simulink model "q_3d_crane"  (Simulink 6.6)
settings: Solver=FixedStepDiscrete  StartTime=0.0  StopTime=inf  FixedStep=0.001  RelTol=1e-3
StopFcn:
  | callback_clear_setpoints
values from neighbouring files (symbols this model uses):
  ALPHA_LIM_ENABLE = 1    [setup_3d_crane.m]
  ALPHA_MAX = 25    [setup_3d_crane.m]
  ALPHA_MIN = - ALPHA_MAX    (= -25)    [setup_3d_crane.m]
  GAMMA_LIM_ENABLE = 1    [setup_3d_crane.m]
  GAMMA_MAX = 25    [setup_3d_crane.m]
  GAMMA_MIN = - GAMMA_MAX    (= -25)    [setup_3d_crane.m]
  IMAX_AMP = 7    [setup_3d_crane.m]
  K_CURR = -2.0    (= -2)    [config_3d_crane.m]
  K_ENC_ALPHA = 2 * pi / (4 * 1024 )    (= 0.00153398078789)    [config_3d_crane.m]
  K_ENC_GAMMA = 2 * pi / (4 * 1024 )    (= 0.00153398078789)    [config_3d_crane.m]
  K_ENC_THETA = 2 * pi / (4 * 1024 ) / Kg_t    (= 1.53398078789e-05)    [config_3d_crane.m]
  K_ENC_X = - Pt / (4 * 1024 ) / Kg_j    [config_3d_crane.m]
  K_ENC_Z = - 2 * pi * r_y_reel / (4 * 1024 ) / Kg_y    [config_3d_crane.m]
  K_J = lqr(A_J,B_J,Q_J,R_J)    [setup_3d_crane.m]
  K_T = lqr(A_T,B_T,Q_T,R_T)    [setup_3d_crane.m]
  Ka = 0.5    [config_3d_crane.m]
  ki = w0^2*p0*(mp*r_y_reel^2+J_phi)/eff_g_y/Kg_y/eff_m_y/Kt_y/r_y_reel    [d_payload_piv_controller.m]
  kp = w0*(2*zeta*p0*J_phi+w0*mp*r_y_reel^2+w0*J_phi+2*zeta*p0*mp*r_y_reel^2)/eff_g_y/Kg_y/eff_m_y/Kt_y/r_y_reel    [d_payload_piv_controller.m]
  kv = (p0*J_phi+2*zeta*w0*mp*r_y_reel^2+2*zeta*w0*J_phi+p0*mp*r_y_reel^2)/eff_g_y/Kg_y/eff_m_y/Kt_y/r_y_reel    [d_payload_piv_controller.m]
  LS_LIM_ENABLE = 1    [setup_3d_crane.m]
  VMAX_DAC = 10    [setup_3d_crane.m]
  wf_gamma = 2 * pi * 2.0    (= 12.5663706144)    [setup_3d_crane.m]
  wf_theta = 2 * pi * 50    (= 314.159265359)    [setup_3d_crane.m]
  wf_x = 2 * pi * 50    (= 314.159265359)    [setup_3d_crane.m]
  wf_z = 2 * pi * 50    (= 314.159265359)    [setup_3d_crane.m]
  X_LIM_ENABLE = 1    [setup_3d_crane.m]
  X_MAX = 0.4    [setup_3d_crane.m]
  X_MIN = - X_MAX    (= -0.4)    [setup_3d_crane.m]
  Z_LIM_ENABLE = 1    [setup_3d_crane.m]
  Z_MAX = 0.7    [setup_3d_crane.m]
  Z_MIN = -0.05    [setup_3d_crane.m]
undefined symbols (not defined in the file or in its folder): DiscIntNeverNeededParam, HIL, qc_get_step_size
libraries: quarc_library x28, simulink x13, simulink_extras x6
settings Model: Creator=MLevis  LastModifiedBy=MLevis  SimulationMode=external  ExtModeTrigDuration=25000
settings SolverCC: PositivePriorityOrder=on
settings RTWCC: SystemTargetFile=quarc_windows.tlc  TemplateMakefile=quarc_default_tmf  Description=QuaRC Win32 Target  ProcessScript=quarc_windows_make_rtw_hook
settings STFCustomTargetCC: TargetFcnLib=ansi_tfl_tmw.mat  TargetPreCompLibLocation=C:\DOCUME~1\ALLUSE~1\APPLIC~1\QUARC\lib\2007a\windows\release  GenFloatMathFcnCalls=ANSI_C  SystemTargetFile=quarc_windows.tlc
settings GRTTargetCC: TargetPreCompLibLocation=C:\DOCUME~1\ALLUSE~1\APPLIC~1\QUARC\lib\2007a\windows\release  MatFileLogging=off  ExtMode=on  ExtModeMexFile=quarc_comm

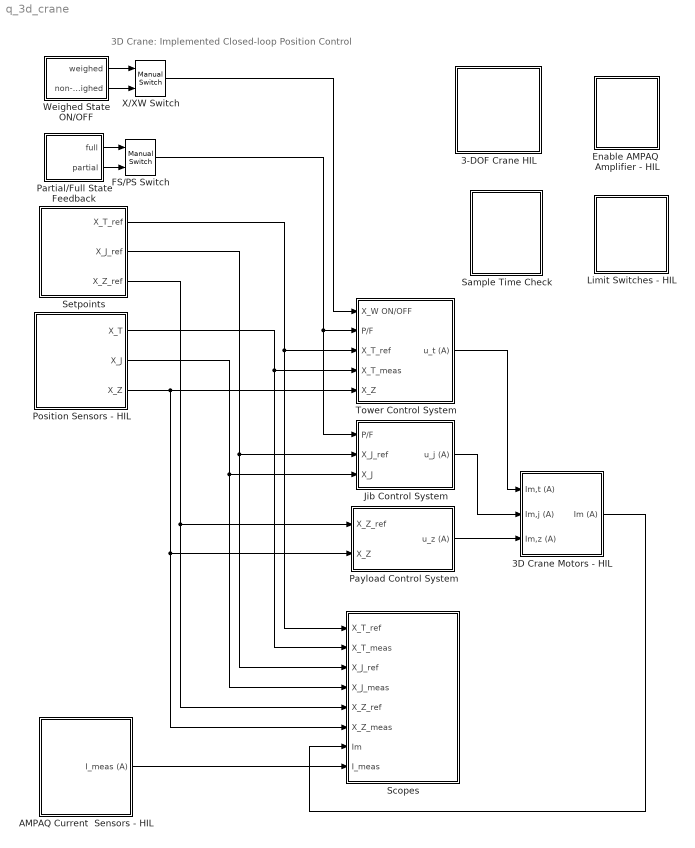
== system q_3d_crane ==
  note: 3D Crane: Implemented Closed-loop Position Control
  3-DOF Crane HIL : Subsystem
  3D Crane Motors - HIL : Subsystem
  AMPAQ Current  Sensors - HIL : Subsystem
  Enable AMPAQ  Amplifier - HIL : Subsystem
  FS/PS Switch : simulink/Signal Routing/Manual Switch  SystemSampleTime=-1  sw=1  action=0  varsize=off
  Jib Control System : Subsystem
  Limit Switches - HIL : Subsystem
  Partial/Full State Feedback : Subsystem
  Payload Control System : Subsystem
  Position Sensors - HIL : Subsystem
  Sample Time Check : Subsystem
  Scopes : Subsystem
  Setpoints : Subsystem
  Tower Control System : Subsystem
  Weighed State ON/OFF : Subsystem
  X/XW Switch : simulink/Signal Routing/Manual Switch  SystemSampleTime=-1  sw=1  action=0  varsize=off
  wires:
  Payload Control System/1(u_z (A)) -> 3D Crane Motors - HIL/3(Im,z (A))
  Tower Control System/1(u_t (A)) -> 3D Crane Motors - HIL/1(Im,t (A))
  Position Sensors - HIL/1(X_T) -> Scopes/2(X_T_meas), Tower Control System/4(X_T_meas)
  Position Sensors - HIL/3(X_Z) -> Scopes/6(X_Z_meas), Payload Control System/2(X_Z), Tower Control System/5(X_Z)
  Position Sensors - HIL/2(X_J) -> Scopes/4(X_J_meas), Jib Control System/3(X_J)
  Setpoints/2(X_J_ref) -> Scopes/3(X_J_ref), Jib Control System/2(X_J_ref)
  Setpoints/1(X_T_ref) -> Scopes/1(X_T_ref), Tower Control System/3(X_T_ref)
  Setpoints/3(X_Z_ref) -> Scopes/5(X_Z_ref), Payload Control System/1(X_Z_ref)
  Jib Control System/1(u_j (A)) -> 3D Crane Motors - HIL/2(Im,j (A))
  Partial/Full State Feedback/1(full) -> FS/PS Switch/1
  Partial/Full State Feedback/2(partial) -> FS/PS Switch/2
  Weighed State ON/OFF/1(weighed) -> X/XW Switch/1
  Weighed State ON/OFF/2(non-weighed) -> X/XW Switch/2
  X/XW Switch/1 -> Tower Control System/1(X_W ON/OFF)
  FS/PS Switch/1 -> Tower Control System/2(P/F), Jib Control System/1(P/F)
  3D Crane Motors - HIL/1(Im (A)) -> Scopes/7(Im)
  AMPAQ Current  Sensors - HIL/1(I_meas (A)) -> Scopes/8(I_meas)

== system q_3d_crane/3-DOF Crane HIL ==
  HIL Initialize : quarc_library/Data Acquisition/Generic/Configuration/HIL Initialize  object_name=HIL-1  board_type=q8  board_number=0  exclusive=off  active=on  hardware_clocks=[0:1]  clock_modes=[0 0]  initial_clock_frequencies=[]  set_clock_params_at_start=on  set_clock_params_at_switch_in=off  set_clock_frequencies_at_start=off  set_clock_frequencies_at_switch_in=off  analog_input_channels=[0:7]  analog_input_maximums=10  analog_input_minimums=-10  set_analog_input_params_at_start=off  set_analog_input_params_at_switch_in=off  analog_output_channels=[0:7]  analog_output_maximums=[10]  analog_output_minimums=[-10]  initial_analog_outputs=[0]  final_analog_outputs=[0]  watchdog_analog_outputs=0  set_analog_output_params_at_start=on  set_analog_output_params_at_switch_in=off  set_analog_outputs_at_start=on  set_analog_outputs_at_switch_in=off  set_analog_outputs_at_terminate=on  set_analog_outputs_at_switch_out=off  set_analog_outputs_on_watchdog=off  digital_input_channels=[]  digital_output_channels=[0:2,4]  digital_output_configuration=[]  initial_digital_outputs=[1]  final_digital_outputs=[1]  watchdog_digital_outputs=[2]  set_digital_output_params_at_start=off  set_digital_output_params_at_switch_in=off  set_digital_outputs_at_start=on  set_digital_outputs_at_switch_in=off  set_digital_outputs_at_terminate=on  set_digital_outputs_at_switch_out=off  set_digital_outputs_on_watchdog=off  encoder_channels=[0:7]  quadrature=[4]  encoder_filter_frequency=(1/120e-9)/1  initial_encoder_counts=[0]  set_encoder_params_at_start=on  set_encoder_params_at_switch_in=off  set_encoder_counts_at_start=on  set_encoder_counts_at_switch_in=off  pwm_channels=[]  pwm_modes=[0]  pwm_frequency=(1/60e-9)/1024  pwm_configuration=[]  pwm_alignment=[]  pwm_polarity=[]  pwm_leading_deadband=[]  pwm_trailing_deadband=[]  initial_pwm_outputs=[0]  final_pwm_outputs=[0]  watchdog_pwm_outputs=[]  set_pwm_params_at_start=on  set_pwm_params_at_switch_in=off  set_pwm_outputs_at_start=on  set_pwm_outputs_at_switch_in=off  set_pwm_outputs_at_terminate=on  set_pwm_outputs_at_switch_out=off  set_pwm_outputs_on_watchdog=off  other_output_channels=[]  initial_other_outputs=[]  final_other_outputs=[]  watchdog_other_outputs=[]  set_other_outputs_at_start=off  set_other_outputs_at_switch_in=off  set_other_outputs_at_terminate=off  set_other_outputs_at_switch_out=off  set_other_outputs_on_watchdog=off
      settings: AttributesFormatString=%<object_name>
  HIL Read Timebase : quarc_library/Data Acquisition/Generic/Timebases/HIL Read Timebase  Tag=unassigned  object_name=HIL-1  clock=0  analog_channels=[0:2]  encoder_channels=[0:4]  digital_channels=[8:12]  other_channels=[]  samples_in_buffer=max(ceil(1/qc_get_step_size), 1)  active=on  vector_output=on  data_type_mode=Inherit via back propagation  encoder_data_type=double  digital_data_type=boolean
  HIL Write : quarc_library/Data Acquisition/Generic/Immediate I//O/HIL Write  Tag=unassigned  object_name=HIL-1  analog_channels=[0:2]  pwm_channels=[]  digital_channels=[0:2,4]  other_channels=[]  sample_time=-1  active=off  vector_input=on
  tag scope: AI=global, DI=global, ENC_CNT=global
  wires:
  HIL Read Timebase/3 -> [DI]
  HIL Read Timebase/1 -> [AI]
  HIL Read Timebase/2 -> [ENC_CNT]
  [DO] -> HIL Write/2
  [AO] -> HIL Write/1

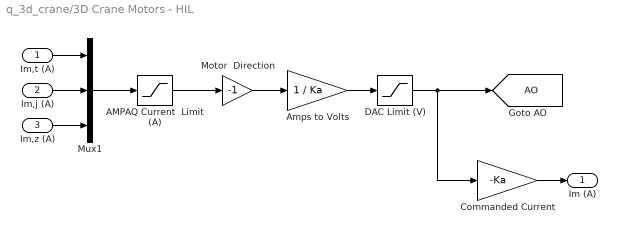
== system q_3d_crane/3D Crane Motors - HIL ==
  Im,t (A) : Inport
  Im,j (A) : Inport  Port=2
  Im,z (A) : Inport  Port=3
  AMPAQ Current  Limit (A) : Saturate  UpperLimit=IMAX_AMP  LowerLimit=-IMAX_AMP
  Amps to Volts : Gain  Gain=1 / Ka  SaturateOnIntegerOverflow=on
  "Commanded Current " : Gain  Gain=-Ka  SaturateOnIntegerOverflow=on
  DAC Limit (V) : Saturate  UpperLimit=VMAX_DAC  LowerLimit=-VMAX_DAC
  Motor  Direction : Gain  Gain=-1
  Mux1 : Mux  Inputs=3
  Im (A) : Outport
  tag scope: AO=global
  wires:
  Amps to Volts/1 -> DAC Limit (V)/1
  DAC Limit (V)/1 -> [AO], "Commanded Current "/1
  AMPAQ Current  Limit (A)/1 -> Motor  Direction/1
  Im,t (A)/1 -> Mux1/1
  Im,j (A)/1 -> Mux1/2
  Im,z (A)/1 -> Mux1/3
  Mux1/1 -> AMPAQ Current  Limit (A)/1
  "Commanded Current "/1 -> Im (A)/1
  Motor  Direction/1 -> Amps to Volts/1

== system q_3d_crane/AMPAQ Current  Sensors - HIL ==
  note: AMPAQ Current Sensors
  Current Sensitivity (A/V) : Gain  Gain=K_CURR
  I_meas (A) : Outport
  wires:
  Current Sensitivity (A/V)/1 -> I_meas (A)/1
  [AI] -> Current Sensitivity (A/V)/1

== system q_3d_crane/Enable AMPAQ  Amplifier - HIL ==
  Enable Amp : Constant  Value=[0 0 0 1]
  tag scope: DO=global
  wires:
  Enable Amp/1 -> [DO]

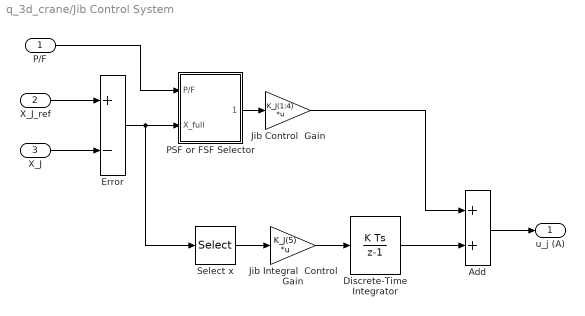
== system q_3d_crane/Jib Control System ==
  P/F : Inport
  X_J_ref : Inport  Port=2
  X_J : Inport  Port=3
  Add : Sum  OutScaling=2^-10
  Discrete-Time Integrator : DiscreteIntegrator  SampleTime=qc_get_step_size  LimitOutput=on  UpperSaturationLimit=2  LowerSaturationLimit=-2  ICPrevOutput=DiscIntNeverNeededParam  ICPrevScaledInput=DiscIntNeverNeededParam
  Error : Sum  Inputs=+-  OutScaling=2^-10
  Jib Control  Gain : Gain  Gain=K_J(1:4)  Multiplication=Matrix(K*u)
  Jib Integral  Control Gain : Gain  Gain=K_J(5)  Multiplication=Matrix(K*u)
  PSF or FSF Selector : Subsystem
  Select x : Selector  IndexOptions=Index vector (dialog)  Indices=1  OutputSizes=1  InputPortWidth=4
  u_j (A) : Outport
  wires:
  PSF or FSF Selector/1(X_out) -> Jib Control  Gain/1
  P/F/1 -> PSF or FSF Selector/1(P/F)
  Add/1 -> u_j (A)/1
  Discrete-Time Integrator/1 -> Add/2
  Jib Control  Gain/1 -> Add/1
  Jib Integral  Control Gain/1 -> Discrete-Time Integrator/1
  Select x/1 -> Jib Integral  Control Gain/1
  X_J/1 -> Error/2
  X_J_ref/1 -> Error/1
  Error/1 -> Select x/1, PSF or FSF Selector/2(X_full)

== system q_3d_crane/Limit Switches - HIL ==
  Constant3 : Constant  Orientation=down  Value=LS_LIM_ENABLE
  Read Limit Switches : Subsystem
  Stop with Limit Switches : Subsystem  TreatAsAtomicUnit=on
  wires:
  Constant3/1 -> Stop with Limit Switches/Enable
  Read Limit Switches/1(tower cw) -> Stop with Limit Switches/1(tower cw)
  Read Limit Switches/2(tower ccw) -> Stop with Limit Switches/2(tower ccw)
  Read Limit Switches/3(jib ret) -> Stop with Limit Switches/3(jib ret)
  Read Limit Switches/4(jib ext) -> Stop with Limit Switches/4(jib ext)
  Read Limit Switches/5(payload max) -> Stop with Limit Switches/5(payload max)

== system q_3d_crane/Partial/Full State Feedback ==
  Full-State : Constant
  Partial-State : Constant  Value=0
  full : Outport
  partial : Outport  Port=2
  wires:
  Full-State/1 -> full/1
  Partial-State/1 -> partial/1

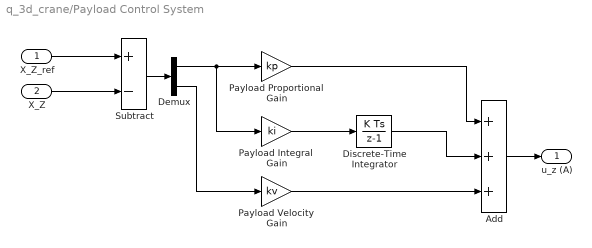
== system q_3d_crane/Payload Control System ==
  X_Z_ref : Inport
  X_Z : Inport  Port=2
  Add : Sum  Inputs=+++  OutScaling=2^-10
  Demux : Demux  Outputs=2
  Discrete-Time Integrator : DiscreteIntegrator  SampleTime=qc_get_step_size  ICPrevOutput=DiscIntNeverNeededParam  ICPrevScaledInput=DiscIntNeverNeededParam
  Payload Integral  Gain : Gain  Gain=ki
  Payload Proportional  Gain : Gain  Gain=kp
  Payload Velocity  Gain : Gain  Gain=kv
  Subtract : Sum  Inputs=+-  OutScaling=2^-10
  u_z (A) : Outport
  wires:
  X_Z/1 -> Subtract/2
  X_Z_ref/1 -> Subtract/1
  Payload Integral  Gain/1 -> Discrete-Time Integrator/1
  Add/1 -> u_z (A)/1
  Payload Proportional  Gain/1 -> Add/1
  Discrete-Time Integrator/1 -> Add/2
  Subtract/1 -> Demux/1
  Demux/1 -> Payload Proportional  Gain/1, Payload Integral  Gain/1
  Demux/2 -> Payload Velocity  Gain/1
  Payload Velocity  Gain/1 -> Add/3

== system q_3d_crane/Position Sensors - HIL ==
  note: 3D Crane Encoders
  Construct Jib State : Subsystem
  Construct Payload State : Subsystem
  Construct Tower State : Subsystem
  Encoder Calibration : Gain  Gain=[K_ENC_THETA, K_ENC_X, K_ENC_Z, K_ENC_ALPHA, K_ENC_GAMMA]
  X_T : Outport
  X_J : Outport  Port=2
  X_Z : Outport  Port=3
  wires:
  [ENC_CNT] -> Encoder Calibration/1
  Encoder Calibration/1 -> Construct Tower State/1(X_read), Construct Jib State/1(X_read), Construct Payload State/1(X_read)
  Construct Tower State/1(X_T) -> X_T/1
  Construct Jib State/1(X_J) -> X_J/1
  Construct Payload State/1(X_Z) -> X_Z/1

== system q_3d_crane/Sample Time Check ==
  Larger than  2x sample time? : simulink/Logic and Bit Operations/Compare To Constant  SystemSampleTime=-1  relop=>  const=2*qc_get_step_size  LogicOutDataTypeMode=uint8  ZeroCross=off
  Max Missed Samples : simulink/Logic and Bit Operations/Compare To Constant  SystemSampleTime=-1  relop=>  const=5  LogicOutDataTypeMode=uint8  ZeroCross=off
  Memory : Memory  Orientation=left
  Sample Time : quarc_library/Sources/Time/Sample Time  Priority=-99  sample_time=qc_get_step_size
  Samples Missed : Display
  Stop with Message : quarc_library/Sinks/Error Handling/Stop with Message  SystemSampleTime=-1  message_type=Fixed error message  message_icon=Error  message=Maximum number of missed samples reached. Please reduce your CPU load.
  Sum : Sum  Inputs=|++
  wires:
  Max Missed Samples/1 -> Stop with Message/1
  Memory/1 -> Sum/2
  Sum/1 -> Memory/1, Max Missed Samples/1, Samples Missed/1
  Larger than  2x sample time?/1 -> Sum/1
  Sample Time/1 -> Larger than  2x sample time?/1

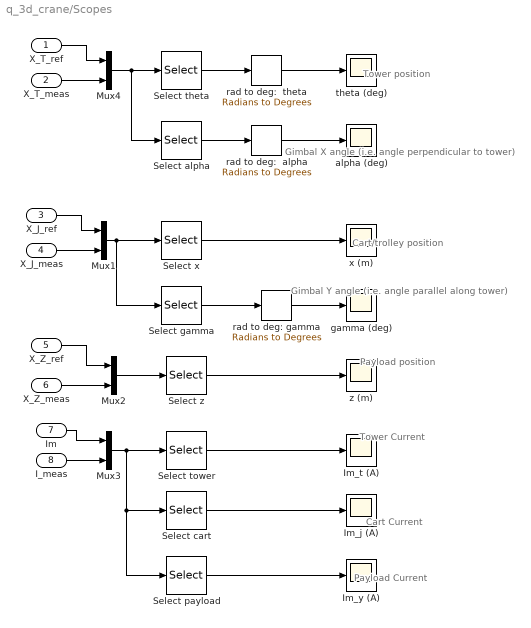
== system q_3d_crane/Scopes ==
  note: Tower Current
  note: Cart Current
  note: Payload Current
  note: Payload position
  note: Cart/trolley position
  note: Tower position
  note: Gimbal X angle
      | (i.e. angle perpendicular to tower)
  note: Gimbal Y angle
      | (i.e. angle parallel along tower)
  X_T_ref : Inport
  X_T_meas : Inport  Port=2
  X_J_ref : Inport  Port=3
  X_J_meas : Inport  Port=4
  X_Z_ref : Inport  Port=5
  X_Z_meas : Inport  Port=6
  Im : Inport  Port=7
  I_meas : Inport  Port=8
  Im_j (A) : Scope
      settings: TimeRange=25  SaveName=ScopeData4
  Im_t (A) : Scope
      settings: TimeRange=25  SaveName=ScopeData3
  Im_y (A) : Scope
      settings: TimeRange=25  SaveName=ScopeData5
  Mux{1..4} (4 alike) : Mux  Inputs=2
  Select alpha : Selector  IndexOptions=Index vector (dialog)  Indices=[2 6]  OutputSizes=1  InputPortWidth=8
  Select cart : Selector  IndexOptions=Index vector (dialog)  Indices=[2 5]  OutputSizes=1  InputPortWidth=6
  Select gamma : Selector  IndexOptions=Index vector (dialog)  Indices=[2 6]  OutputSizes=1  InputPortWidth=8
  Select payload : Selector  IndexOptions=Index vector (dialog)  Indices=[3 6]  OutputSizes=1  InputPortWidth=6
  Select theta : Selector  IndexOptions=Index vector (dialog)  Indices=[1 5]  OutputSizes=1  InputPortWidth=8
  Select tower : Selector  IndexOptions=Index vector (dialog)  Indices=[1 4]  OutputSizes=1  InputPortWidth=6
  Select x : Selector  IndexOptions=Index vector (dialog)  Indices=[1 5]  OutputSizes=1  InputPortWidth=8
  Select z : Selector  IndexOptions=Index vector (dialog)  Indices=[1 3]  OutputSizes=1  InputPortWidth=4
  alpha (deg) : Scope
      settings: TimeRange=25  YMin=-15  YMax=15
  gamma (deg) : Scope
      settings: TimeRange=25  SaveName=ScopeData9
  rad to deg:  theta : simulink_extras/Transformations/Radians to Degrees  SystemSampleTime=-1
  rad to deg: gamma : simulink_extras/Transformations/Radians to Degrees  SystemSampleTime=-1
  rad to deg:  alpha : simulink_extras/Transformations/Radians to Degrees  SystemSampleTime=-1
  theta (deg) : Scope
      settings: TimeRange=25  YMin=-150  YMax=150  SaveName=ScopeData8
  x (m) : Scope
      settings: TimeRange=25  YMin=-1  YMax=1
  z (m) : Scope
      settings: TimeRange=25  YMin=0  YMax=0.65  SaveName=ScopeData2
  wires:
  I_meas/1 -> Mux3/2
  Mux3/1 -> Select tower/1, Select payload/1, Select cart/1
  Im/1 -> Mux3/1
  rad to deg:  theta/1 -> theta (deg)/1
  rad to deg: gamma/1 -> gamma (deg)/1
  rad to deg:  alpha/1 -> alpha (deg)/1
  Select theta/1 -> rad to deg:  theta/1
  X_T_ref/1 -> Mux4/1
  Mux4/1 -> Select theta/1, Select alpha/1
  Select x/1 -> x (m)/1
  Mux2/1 -> Select z/1
  Select alpha/1 -> rad to deg:  alpha/1
  Select gamma/1 -> rad to deg: gamma/1
  X_J_ref/1 -> Mux1/1
  X_J_meas/1 -> Mux1/2
  Mux1/1 -> Select x/1, Select gamma/1
  X_Z_ref/1 -> Mux2/1
  X_Z_meas/1 -> Mux2/2
  Select z/1 -> z (m)/1
  X_T_meas/1 -> Mux4/2
  Select tower/1 -> Im_t (A)/1
  Select cart/1 -> Im_j (A)/1
  Select payload/1 -> Im_y (A)/1

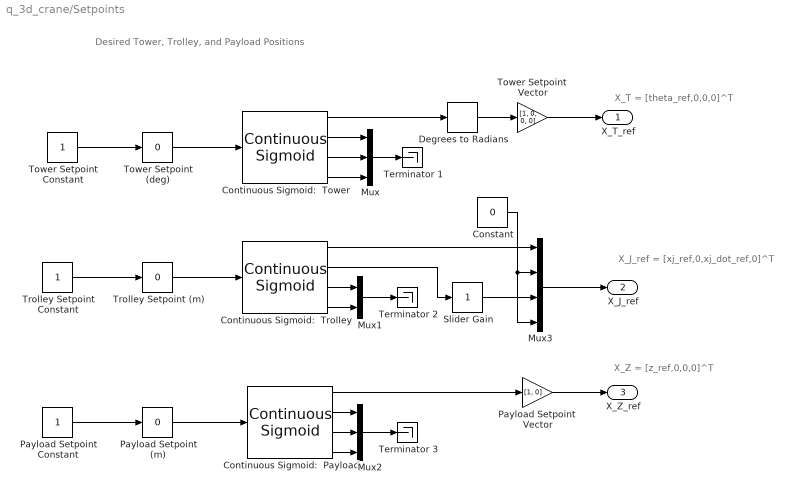
== system q_3d_crane/Setpoints ==
  note: X_J_ref = [xj_ref,0,xj_dot_ref,0]^T
  note: X_T = [theta_ref,0,0,0]^T
  note: X_Z = [z_ref,0,0,0]^T
  note: Desired Tower, Trolley, and Payload Positions
  Constant : Constant  Value=0
  Continuous Sigmoid:  Payload : quarc_library/Sources/Sigmoids/Continuous Sigmoid  params_source=Internal (dialog parameters)  max_velocity=0.25  max_acceleration=0.25  initial_position=0  initial_velocity=0  hold_off=0.5  input_sample_time=-1  output_sample_time=qc_get_step_size
  Continuous Sigmoid:  Tower : quarc_library/Sources/Sigmoids/Continuous Sigmoid  params_source=Internal (dialog parameters)  max_velocity=75  max_acceleration=45  initial_position=0  initial_velocity=0  hold_off=0.5  input_sample_time=-1  output_sample_time=qc_get_step_size
  Continuous Sigmoid:  Trolley : quarc_library/Sources/Sigmoids/Continuous Sigmoid  params_source=Internal (dialog parameters)  max_velocity=0.75  max_acceleration=1.5  initial_position=0  initial_velocity=0  hold_off=0.5  input_sample_time=-1  output_sample_time=qc_get_step_size
  Degrees to Radians : simulink_extras/Transformations/Degrees to Radians  SystemSampleTime=-1
  Mux : Mux  Inputs=3
  Mux1 : Mux  Inputs=2
  Mux2 : Mux  Inputs=3
  Mux3 : Mux
  "Payload Setpoint Constant " : Constant
  Payload Setpoint  Vector : Gain  Gain=[1, 0]
  Payload Setpoint (m) : simulink/Math Operations/Slider Gain  SystemSampleTime=-1  low=0  gain=0  high=0.8
  Slider Gain : simulink/Math Operations/Slider Gain  SystemSampleTime=-1  low=0  gain=1  high=1
  Terminator 1 : Terminator
  Terminator 2 : Terminator
  Terminator 3 : Terminator
  "Tower Setpoint Constant " : Constant
  Tower Setpoint  Vector : Gain  Gain=[1, 0, 0, 0]
  Tower Setpoint (deg) : simulink/Math Operations/Slider Gain  SystemSampleTime=-1  low=-120  gain=0  high=120
  "Trolley Setpoint Constant " : Constant
  Trolley Setpoint (m) : simulink/Math Operations/Slider Gain  SystemSampleTime=-1  low=-0.2  gain=0  high=0.2
  X_T_ref : Outport
  X_J_ref : Outport  Port=2
  X_Z_ref : Outport  Port=3
  wires:
  Continuous Sigmoid:  Tower/1 -> Degrees to Radians/1
  "Tower Setpoint Constant "/1 -> Tower Setpoint (deg)/1
  Tower Setpoint (deg)/1 -> Continuous Sigmoid:  Tower/1
  "Trolley Setpoint Constant "/1 -> Trolley Setpoint (m)/1
  "Payload Setpoint Constant "/1 -> Payload Setpoint (m)/1
  Degrees to Radians/1 -> Tower Setpoint  Vector/1
  Continuous Sigmoid:  Tower/2 -> Mux/1
  Continuous Sigmoid:  Tower/3 -> Mux/2
  Continuous Sigmoid:  Tower/4 -> Mux/3
  Mux/1 -> Terminator 1/1
  Payload Setpoint (m)/1 -> Continuous Sigmoid:  Payload/1
  Tower Setpoint  Vector/1 -> X_T_ref/1
  Continuous Sigmoid:  Payload/1 -> Payload Setpoint  Vector/1
  Payload Setpoint  Vector/1 -> X_Z_ref/1
  Trolley Setpoint (m)/1 -> Continuous Sigmoid:  Trolley/1
  Mux3/1 -> X_J_ref/1
  Continuous Sigmoid:  Trolley/1 -> Mux3/1
  Constant/1 -> Mux3/2, Mux3/4
  Continuous Sigmoid:  Trolley/2 -> Slider Gain/1
  Slider Gain/1 -> Mux3/3
  Mux1/1 -> Terminator 2/1
  Mux2/1 -> Terminator 3/1
  Continuous Sigmoid:  Payload/2 -> Mux2/1
  Continuous Sigmoid:  Payload/3 -> Mux2/2
  Continuous Sigmoid:  Payload/4 -> Mux2/3
  Continuous Sigmoid:  Trolley/3 -> Mux1/1
  Continuous Sigmoid:  Trolley/4 -> Mux1/2

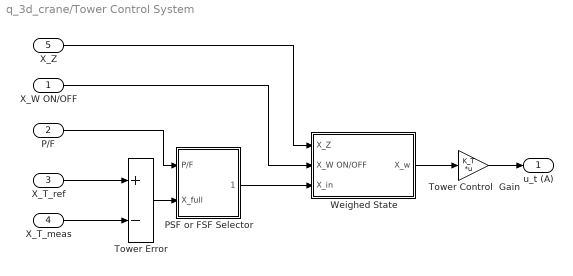
== system q_3d_crane/Tower Control System ==
  X_W ON/OFF : Inport
  P/F : Inport  Port=2
  X_T_ref : Inport  Port=3
  X_T_meas : Inport  Port=4
  X_Z : Inport  Port=5
  PSF or FSF Selector : Subsystem
  Tower Control  Gain : Gain  Gain=K_T  Multiplication=Matrix(K*u)
  Tower Error : Sum  Inputs=+-  OutScaling=2^-10
  Weighed State : Subsystem
  u_t (A) : Outport
  wires:
  Tower Control  Gain/1 -> u_t (A)/1
  X_T_ref/1 -> Tower Error/1
  X_T_meas/1 -> Tower Error/2
  P/F/1 -> PSF or FSF Selector/1(P/F)
  Tower Error/1 -> PSF or FSF Selector/2(X_full)
  X_Z/1 -> Weighed State/1(X_Z)
  X_W ON/OFF/1 -> Weighed State/2(X_W ON/OFF)
  PSF or FSF Selector/1(X_out) -> Weighed State/3(X_in)
  Weighed State/1(X_w) -> Tower Control  Gain/1

== system q_3d_crane/Weighed State ON/OFF ==
  Full State : Constant  Value=0
  Weighed State : Constant
  weighed : Outport
  non-weighed : Outport  Port=2
  wires:
  Weighed State/1 -> weighed/1
  Full State/1 -> non-weighed/1

== system q_3d_crane/Jib Control System/PSF or FSF Selector ==
  note: Partial-state or Full-state Feedback
  note: 0 = partial and 1 = full,
  note: state
  note: control input
  P/F : Inport
  X_full : Inport  Port=2
  Constant: FS : Constant  Value=[1 1 1 1]
  Constant: PS : Constant  Value=[1 0 1 0]
  Full-state : Product  RndMeth=Zero
  Multiport Switch : MultiPortSwitch  Inputs=2  zeroidx=on
  Partial-state : Product  RndMeth=Zero
  X_out : Outport
  wires:
  Constant: FS/1 -> Full-state/2
  Constant: PS/1 -> Partial-state/1
  Partial-state/1 -> Multiport Switch/2
  Full-state/1 -> Multiport Switch/3
  Multiport Switch/1 -> X_out/1
  P/F/1 -> Multiport Switch/1
  X_full/1 -> Partial-state/2, Full-state/1

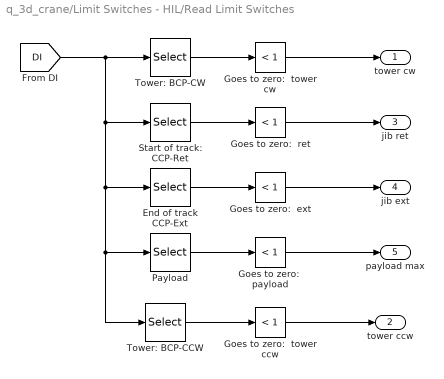
== system q_3d_crane/Limit Switches - HIL/Read Limit Switches ==
  End of track CCP-Ext : Selector  IndexOptions=Index vector (dialog)  Indices=3  OutputSizes=1  InputPortWidth=5
  Goes to zero:  ext : simulink/Logic and Bit Operations/Compare To Constant  SystemSampleTime=-1  relop=<  const=1  LogicOutDataTypeMode=uint8  ZeroCross=off
  Goes to zero:  payload : simulink/Logic and Bit Operations/Compare To Constant  SystemSampleTime=-1  relop=<  const=1  LogicOutDataTypeMode=uint8  ZeroCross=off
  Goes to zero:  ret : simulink/Logic and Bit Operations/Compare To Constant  SystemSampleTime=-1  relop=<  const=1  LogicOutDataTypeMode=uint8  ZeroCross=off
  Goes to zero:  tower ccw : simulink/Logic and Bit Operations/Compare To Constant  SystemSampleTime=-1  relop=<  const=1  LogicOutDataTypeMode=uint8  ZeroCross=off
  Goes to zero:  tower cw : simulink/Logic and Bit Operations/Compare To Constant  SystemSampleTime=-1  relop=<  const=1  LogicOutDataTypeMode=uint8  ZeroCross=off
  Payload : Selector  IndexOptions=Index vector (dialog)  Indices=4  OutputSizes=1  InputPortWidth=5
  Start of track: CCP-Ret : Selector  IndexOptions=Index vector (dialog)  Indices=2  OutputSizes=1  InputPortWidth=5
  Tower: BCP-CCW : Selector  IndexOptions=Index vector (dialog)  Indices=5  OutputSizes=1  InputPortWidth=5
  Tower: BCP-CW : Selector  IndexOptions=Index vector (dialog)  Indices=1  OutputSizes=1  InputPortWidth=5
  tower cw : Outport
  tower ccw : Outport  Port=2
  jib ret : Outport  Port=3
  jib ext : Outport  Port=4
  payload max : Outport  Port=5
  wires:
  Goes to zero:  tower ccw/1 -> tower ccw/1
  Tower: BCP-CCW/1 -> Goes to zero:  tower ccw/1
  End of track CCP-Ext/1 -> Goes to zero:  ext/1
  Start of track: CCP-Ret/1 -> Goes to zero:  ret/1
  Goes to zero:  ext/1 -> jib ext/1
  Goes to zero:  ret/1 -> jib ret/1
  Tower: BCP-CW/1 -> Goes to zero:  tower cw/1
  Goes to zero:  tower cw/1 -> tower cw/1
  Goes to zero:  payload/1 -> payload max/1
  Payload/1 -> Goes to zero:  payload/1
  [DI] -> Tower: BCP-CW/1, Start of track: CCP-Ret/1, Tower: BCP-CCW/1, Payload/1, End of track CCP-Ext/1

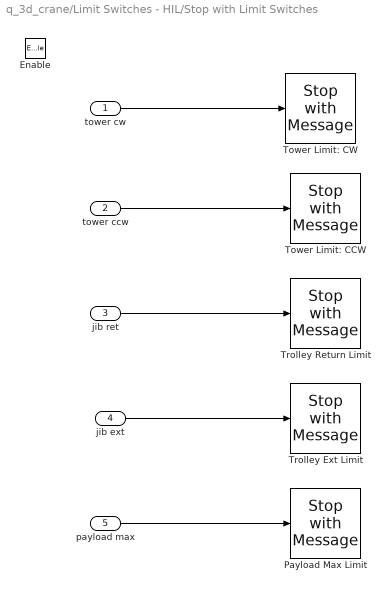
== system q_3d_crane/Limit Switches - HIL/Stop with Limit Switches ==
  tower cw : Inport
  tower ccw : Inport  Port=2
  jib ret : Inport  Port=3
  jib ext : Inport  Port=4
  payload max : Inport  Port=5
  Enable : EnablePort
  Payload Max Limit : quarc_library/Sinks/Error Handling/Stop with Message  SystemSampleTime=-1  message_type=Fixed error message  message_icon=Error  message=Payload limit switch triggered: payload at max height.
  Tower Limit: CCW : quarc_library/Sinks/Error Handling/Stop with Message  SystemSampleTime=-1  message_type=Fixed error message  message_icon=Error  message=Tower limit switch triggered: tower reached max counter-clockwise angle.
  Tower Limit: CW : quarc_library/Sinks/Error Handling/Stop with Message  SystemSampleTime=-1  message_type=Fixed error message  message_icon=Error  message=Tower limit switch triggered: tower reached max clockwise angle.
  Trolley Ext Limit : quarc_library/Sinks/Error Handling/Stop with Message  SystemSampleTime=-1  message_type=Fixed error message  message_icon=Error  message=EXT limit switch triggered: trolley at max position.
  Trolley Return Limit : quarc_library/Sinks/Error Handling/Stop with Message  SystemSampleTime=-1  message_type=Fixed error message  message_icon=Error  message=RET limit switch triggered: trolley at min position.
  wires:
  tower cw/1 -> Tower Limit: CW/1
  jib ret/1 -> Trolley Return Limit/1
  jib ext/1 -> Trolley Ext Limit/1
  payload max/1 -> Payload Max Limit/1
  tower ccw/1 -> Tower Limit: CCW/1

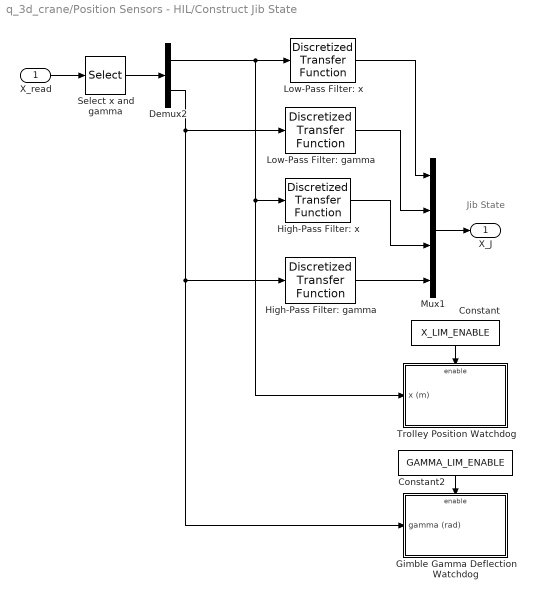
== system q_3d_crane/Position Sensors - HIL/Construct Jib State ==
  note: Jib State
  X_read : Inport
  Constant : Constant  Orientation=down  Value=X_LIM_ENABLE
  Constant2 : Constant  Orientation=down  Value=GAMMA_LIM_ENABLE
  Demux2 : Demux  Outputs=2
  Gimble Gamma Deflection Watchdog : Subsystem  TreatAsAtomicUnit=on
  High-Pass Filter: gamma : quarc_library/Discrete/Discretized Transfer Function  SystemSampleTime=-1  num=[wf_gamma 0]  den=[1 wf_gamma]  method=tustin  Ts=qc_get_step_size
  High-Pass Filter: x : quarc_library/Discrete/Discretized Transfer Function  SystemSampleTime=-1  num=[wf_x 0]  den=[1 wf_x]  method=tustin  Ts=qc_get_step_size
  Low-Pass Filter: gamma : quarc_library/Discrete/Discretized Transfer Function  SystemSampleTime=-1  num=[wf_gamma]  den=[1 wf_gamma]  method=tustin  Ts=qc_get_step_size
  Low-Pass Filter: x : quarc_library/Discrete/Discretized Transfer Function  SystemSampleTime=-1  num=[wf_x]  den=[1 wf_x]  method=tustin  Ts=qc_get_step_size
  Mux1 : Mux
  Select x and gamma : Selector  IndexOptions=Index vector (dialog)  Indices=[2, 5]  OutputSizes=1  InputPortWidth=5
  Trolley Position Watchdog : Subsystem  TreatAsAtomicUnit=on
  X_J : Outport
  wires:
  Constant/1 -> Trolley Position Watchdog/Enable
  Mux1/1 -> X_J/1
  Select x and gamma/1 -> Demux2/1
  Constant2/1 -> Gimble Gamma Deflection Watchdog/Enable
  X_read/1 -> Select x and gamma/1
  Demux2/1 -> Trolley Position Watchdog/1(x (m)), High-Pass Filter: x/1, Low-Pass Filter: x/1
  Demux2/2 -> Gimble Gamma Deflection Watchdog/1(gamma (rad)), High-Pass Filter: gamma/1, Low-Pass Filter: gamma/1
  Low-Pass Filter: x/1 -> Mux1/1
  Low-Pass Filter: gamma/1 -> Mux1/2
  High-Pass Filter: x/1 -> Mux1/3
  High-Pass Filter: gamma/1 -> Mux1/4

== system q_3d_crane/Position Sensors - HIL/Construct Payload State ==
  note: Payload State
  X_read : Inport
  Constant3 : Constant  Orientation=down  Value=Z_LIM_ENABLE
  High-Pass Filter: z : quarc_library/Discrete/Discretized Transfer Function  SystemSampleTime=-1  num=[wf_z 0]  den=[1 wf_z]  method=tustin  Ts=qc_get_step_size
  Mux2 : Mux  Inputs=2
  Payload Position Watchdog : Subsystem  TreatAsAtomicUnit=on
  Select z : Selector  IndexOptions=Index vector (dialog)  Indices=3  OutputSizes=1  InputPortWidth=5
  X_Z : Outport
  wires:
  Select z/1 -> Mux2/1, Payload Position Watchdog/1(z (m)), High-Pass Filter: z/1
  Mux2/1 -> X_Z/1
  Constant3/1 -> Payload Position Watchdog/Enable
  X_read/1 -> Select z/1
  High-Pass Filter: z/1 -> Mux2/2

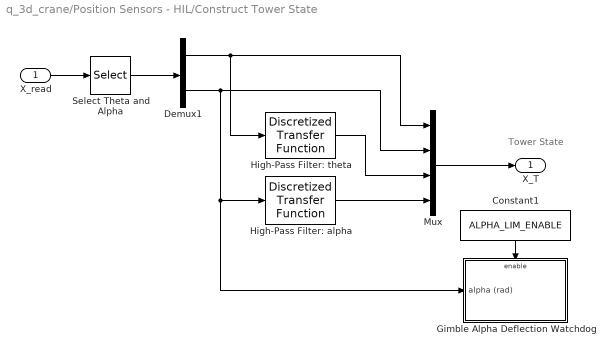
== system q_3d_crane/Position Sensors - HIL/Construct Tower State ==
  note: Tower State
  X_read : Inport
  Constant1 : Constant  Orientation=down  Value=ALPHA_LIM_ENABLE
  Demux1 : Demux  Outputs=2
  Gimble Alpha Deflection Watchdog : Subsystem  TreatAsAtomicUnit=on
  High-Pass Filter: alpha : quarc_library/Discrete/Discretized Transfer Function  SystemSampleTime=-1  num=[wf_gamma 0]  den=[1 wf_gamma]  method=tustin  Ts=qc_get_step_size
  High-Pass Filter: theta : quarc_library/Discrete/Discretized Transfer Function  SystemSampleTime=-1  num=[wf_theta 0]  den=[1 wf_theta]  method=tustin  Ts=qc_get_step_size
  Mux : Mux
  Select Theta and Alpha : Selector  IndexOptions=Index vector (dialog)  Indices=[1, 4]  OutputSizes=1  InputPortWidth=5
  X_T : Outport
  wires:
  Constant1/1 -> Gimble Alpha Deflection Watchdog/Enable
  Mux/1 -> X_T/1
  Select Theta and Alpha/1 -> Demux1/1
  X_read/1 -> Select Theta and Alpha/1
  Demux1/1 -> Mux/1, High-Pass Filter: theta/1
  Demux1/2 -> Mux/2, Gimble Alpha Deflection Watchdog/1(alpha (rad)), High-Pass Filter: alpha/1
  High-Pass Filter: theta/1 -> Mux/3
  High-Pass Filter: alpha/1 -> Mux/4

== system q_3d_crane/Tower Control System/PSF or FSF Selector ==
  note: control input
  note: state
  note: 0 = partial and 1 = full,
  note: Partial-state or Full-state Feedback
  P/F : Inport
  X_full : Inport  Port=2
  Constant: FS : Constant  Value=[1 1 1 1]
  Constant: PS : Constant  Value=[1 0 1 0]
  Full-state : Product  RndMeth=Zero
  Multiport Switch : MultiPortSwitch  Inputs=2  zeroidx=on
  Partial-state : Product  RndMeth=Zero
  X_out : Outport
  wires:
  X_full/1 -> Full-state/1, Partial-state/2
  P/F/1 -> Multiport Switch/1
  Multiport Switch/1 -> X_out/1
  Full-state/1 -> Multiport Switch/3
  Partial-state/1 -> Multiport Switch/2
  Constant: PS/1 -> Partial-state/1
  Constant: FS/1 -> Full-state/2

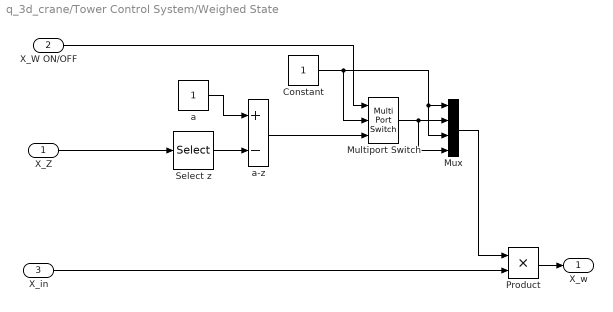
== system q_3d_crane/Tower Control System/Weighed State ==
  X_Z : Inport
  X_W ON/OFF : Inport  Port=2
  X_in : Inport  Port=3
  Constant : Constant
  Multiport Switch : MultiPortSwitch  Inputs=2  zeroidx=on
  Mux : Mux
  Product : Product  RndMeth=Zero
  Select z : Selector  IndexOptions=Index vector (dialog)  Indices=1  OutputSizes=1  InputPortWidth=2
  a : Constant
  a-z : Sum  Inputs=+-  OutScaling=2^-10
  X_w : Outport
  wires:
  X_in/1 -> Product/2
  Product/1 -> X_w/1
  X_Z/1 -> Select z/1
  Select z/1 -> a-z/2
  a-z/1 -> Multiport Switch/3
  Constant/1 -> Mux/1, Mux/3, Multiport Switch/2
  a/1 -> a-z/1
  X_W ON/OFF/1 -> Multiport Switch/1
  Multiport Switch/1 -> Mux/4, Mux/2
  Mux/1 -> Product/1

== system q_3d_crane/Position Sensors - HIL/Construct Jib State/Gimble Gamma Deflection Watchdog ==
  gamma (rad) : Inport
  Enable : EnablePort
  Check Maximum Allowed Angle : RelationalOperator  Operator=<  InputSameDT=on
  Check Minimum Allowed Angle : RelationalOperator  Operator=<  InputSameDT=on
  Max Gamma : quarc_library/Sinks/Error Handling/Stop with Message  SystemSampleTime=-1  message_type=Fixed error message  message_icon=Error  message=Maximum gamma gimble angle reached.
  Min Gamma : quarc_library/Sinks/Error Handling/Stop with Message  SystemSampleTime=-1  message_type=Fixed error message  message_icon=Error  message=Minimum gamma gimble angle reached.
  Radians to Degrees : simulink_extras/Transformations/Radians to Degrees  SystemSampleTime=-1
  X MAX : Constant  Value=GAMMA_MAX
  X MIN : Constant  Value=GAMMA_MIN
  wires:
  X MAX/1 -> Check Maximum Allowed Angle/1
  Check Minimum Allowed Angle/1 -> Min Gamma/1
  X MIN/1 -> Check Minimum Allowed Angle/2
  gamma (rad)/1 -> Radians to Degrees/1
  Check Maximum Allowed Angle/1 -> Max Gamma/1
  Radians to Degrees/1 -> Check Maximum Allowed Angle/2, Check Minimum Allowed Angle/1

== system q_3d_crane/Position Sensors - HIL/Construct Jib State/Trolley Position Watchdog ==
  x (m) : Inport
  Enable : EnablePort
  Check Maximum Allowed Position : RelationalOperator  Operator=<  InputSameDT=on
  Check Minimum Allowed Position : RelationalOperator  Operator=<  InputSameDT=on
  Max Trolley : quarc_library/Sinks/Error Handling/Stop with Message  SystemSampleTime=-1  message_type=Fixed error message  message_icon=Error  message=Maximum trolley position reached.
  Min Trolley : quarc_library/Sinks/Error Handling/Stop with Message  SystemSampleTime=-1  message_type=Fixed error message  message_icon=Error  message=Minimum trolley position reached.
  X IN : Constant  Value=X_MIN
  X MAX : Constant  Value=X_MAX
  wires:
  Check Maximum Allowed Position/1 -> Max Trolley/1
  x (m)/1 -> Check Minimum Allowed Position/1, Check Maximum Allowed Position/2
  X IN/1 -> Check Minimum Allowed Position/2
  Check Minimum Allowed Position/1 -> Min Trolley/1
  X MAX/1 -> Check Maximum Allowed Position/1

== system q_3d_crane/Position Sensors - HIL/Construct Payload State/Payload Position Watchdog ==
  z (m) : Inport
  Enable : EnablePort
  Check Maximum Allowed Position : RelationalOperator  Operator=<  InputSameDT=on
  Check Minimum Allowed Position : RelationalOperator  Operator=<  InputSameDT=on
  Max Payload Position : quarc_library/Sinks/Error Handling/Stop with Message  SystemSampleTime=-1  message_type=Fixed error message  message_icon=Error  message=Maximum payload position reached.
  Min Payload Position : quarc_library/Sinks/Error Handling/Stop with Message  SystemSampleTime=-1  message_type=Fixed error message  message_icon=Error  message=Minimum payload position reached.
  X IN : Constant  Value=Z_MIN
  X MAX : Constant  Value=Z_MAX
  wires:
  X MAX/1 -> Check Maximum Allowed Position/1
  Check Minimum Allowed Position/1 -> Min Payload Position/1
  X IN/1 -> Check Minimum Allowed Position/2
  z (m)/1 -> Check Maximum Allowed Position/2, Check Minimum Allowed Position/1
  Check Maximum Allowed Position/1 -> Max Payload Position/1

== system q_3d_crane/Position Sensors - HIL/Construct Tower State/Gimble Alpha Deflection Watchdog ==
  alpha (rad) : Inport
  Enable : EnablePort
  Check Maximum Allowed Angle : RelationalOperator  Operator=<  InputSameDT=on
  Check Minimum Allowed Angle : RelationalOperator  Operator=<  InputSameDT=on
  Max Alpha : quarc_library/Sinks/Error Handling/Stop with Message  SystemSampleTime=-1  message_type=Fixed error message  message_icon=Error  message=Maximum alpha gimble angle reached.
  Min Angle : quarc_library/Sinks/Error Handling/Stop with Message  SystemSampleTime=-1  message_type=Fixed error message  message_icon=Error  message=Minimum alpha gimble angle reached.
  Radians to Degrees : simulink_extras/Transformations/Radians to Degrees  SystemSampleTime=-1
  X MAX : Constant  Value=ALPHA_MAX
  X MIN : Constant  Value=ALPHA_MIN
  wires:
  Radians to Degrees/1 -> Check Minimum Allowed Angle/1, Check Maximum Allowed Angle/2
  Check Maximum Allowed Angle/1 -> Max Alpha/1
  alpha (rad)/1 -> Radians to Degrees/1
  X MIN/1 -> Check Minimum Allowed Angle/2
  Check Minimum Allowed Angle/1 -> Min Angle/1
  X MAX/1 -> Check Maximum Allowed Angle/1
